simulink model "modelR2016bMAC"  (R2016b)
settings: Solver=VariableStepAuto  StartTime=0.0  StopTime=time  FixedStep=0.02  RelTol=1e-3  EnableMultiTasking=on
InitFcn:
  | m
StopFcn:
  | plotting
undefined symbols (not defined in the file): Aw, Awi, B, CurrentEnabled, D, E, e0, Eta0, g, Gi, Gpd, H, HiPAPpeaksEnabled, Is, Lambda, M, N, Omega, P0, path, Q, R, SensNoiseEnabled, T, tau_max, tau_min, Tb, WavesEnabled, x0
settings Model: Creator=Gaspar  LastModifiedBy=sbuadu
settings DataIOCC: LimitDataPoints=on  SaveFormat=Structure  SaveOutput=off  SaveTime=off
settings OptimizationCC: DefaultParameterBehavior=Inlined  LifeSpan=inf
settings DebuggingCC: UnderspecifiedInitializationDetection=Classic  MergeDetectMultiDrivingBlocksExec=none  SFUnexpectedBacktrackingDiag=warning  SFNoUnconditionalDefaultTransitionDiag=warning  SFExecutionAtInitializationDiag=none
settings GRTTargetCC: TargetLangStandard=C89/C90 (ANSI)
settings ConfigComp: CovMetricSettings=dw  CovHtmlReporting=on  CovSaveCumulativeToWorkspaceVar=on  CovSaveSingleToWorkspaceVar=on  CovExternalEMLEnable=off

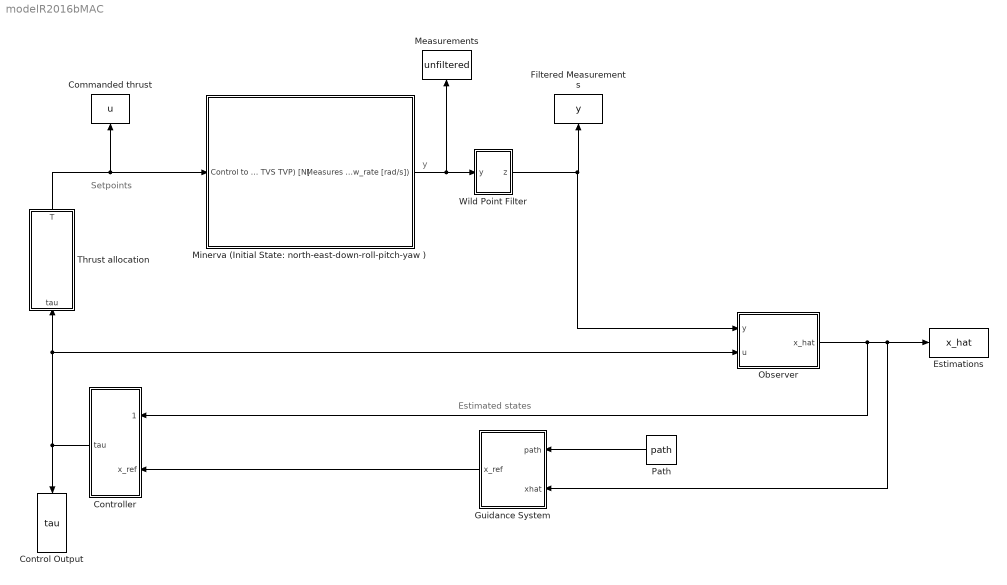
== system modelR2016bMAC ==
  note: Estimated states
  note: y
  note: Setpoints
  Commanded thrust : ToWorkspace  VariableName=u  SaveFormat=Timeseries  SampleTime=T
  Control Output : ToWorkspace  VariableName=tau  SaveFormat=Timeseries  SampleTime=-1
  Controller : Subsystem
  Estimations : ToWorkspace  VariableName=x_hat  SaveFormat=Timeseries  SampleTime=T
  Filtered Measurements : ToWorkspace  VariableName=y  SaveFormat=Timeseries  SampleTime=T
  Guidance System : Subsystem
  Measurements : ToWorkspace  VariableName=unfiltered  SaveFormat=Timeseries  SampleTime=T
  Minerva (Initial State: north-east-down-roll-pitch-yaw ) : Subsystem  mask{sfcnParam1=CurrentEnabled, sfcnParam2=Eta0, sfcnParam3=HiPAPpeaksEnabled, sfcnParam4=SensNoiseEnabled, sfcnParam5=WavesEnabled}
      mask prompts: sfcnParam1 "CurrentEnabled:"; sfcnParam2 "Eta0:"; sfcnParam3 "HiPAPpeaksEnabled:"; sfcnParam4 "SensNoiseEnabled:"; sfcnParam5 "WavesEnabled:"
      mask help: Simulink:masks:GenSFuncDesc_MD
      mask Help: eval('feval(''rtwprivate'',''rtwhelpview'',''rtw_sfcn_block'')');
      mask Display: image(imread(strcat(cd,'/ROVMinerva.jpg'),'jpg'),'center')
  Observer : Subsystem
  "Path " : Constant  Value=path  SampleTime=T
  "Thrust allocation " : Subsystem
  Wild Point Filter : Subsystem
  wires:
  Wild Point Filter/1(z) -> Observer/1(y), Filtered Measurements/1
  Minerva (Initial State: north-east-down-roll-pitch-yaw )/1(Measures (n[m] e[m] d[m] heading [rad] yaw_rate [rad/s])) -> Measurements/1, Wild Point Filter/1(y)
  "Thrust allocation "/1(T) -> Minerva (Initial State: north-east-down-roll-pitch-yaw )/1(Control to Thrusters (THS THP THL TVS TVP) [N]), Commanded thrust/1
  Controller/1(tau) -> Observer/2(u), "Thrust allocation "/1(tau), Control Output/1
  Observer/1(x_hat) -> Controller/1(x_hat), Guidance System/2("xhat "), Estimations/1
  "Path "/1 -> Guidance System/1(path)
  Guidance System/1(x_ref) -> Controller/2(x_ref)

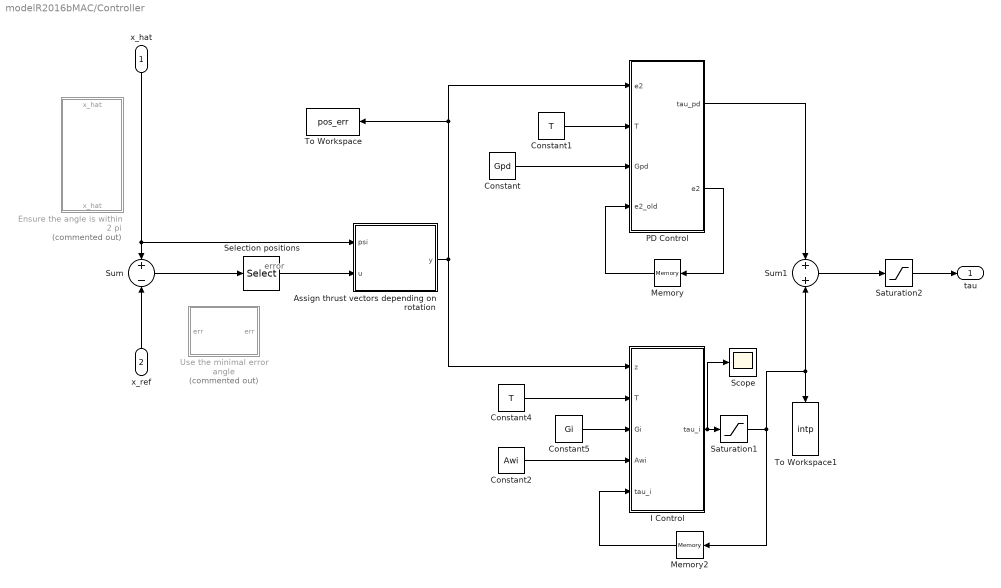
== system modelR2016bMAC/Controller ==
  note: error
  x_hat : Inport  PortDimensions=[20,1]  SampleTime=T
  x_ref : Inport  Port=2  PortDimensions=[20,1]  SampleTime=T
  Assign thrust vectors depending on rotation : MATLAB Function  TreatAsAtomicUnit=on
  Constant : Constant  Value=Gpd  SampleTime=T
  Constant1 : Constant  Value=T  SampleTime=T
  Constant2 : Constant  Value=Awi  SampleTime=T
  Constant4 : Constant  Value=T  SampleTime=T
  Constant5 : Constant  Value=Gi  SampleTime=T
  Ensure the angle is within 2 pi : MATLAB Function  Commented=on  TreatAsAtomicUnit=on
  I Control : MATLAB Function  TreatAsAtomicUnit=on
  Memory : Memory  X0=e0  InheritSampleTime=on
  Memory2 : Memory  X0=e0  InheritSampleTime=on
  PD Control : MATLAB Function  TreatAsAtomicUnit=on
  Saturation1 : Saturate  UpperLimit=Is*tau_max  LowerLimit=Is*tau_min
  Saturation2 : Saturate  UpperLimit=tau_max  LowerLimit=tau_min
  Scope : Scope
  Selection positions : Selector  InputPortWidth=20  IndexOptions=Index vector (dialog)  Indices=[9:12]  OutputSizes=1
  Sum : Sum  Inputs=+-
  Sum1 : Sum
  To Workspace : ToWorkspace  VariableName=pos_err  SaveFormat=Timeseries  SampleTime=T
  To Workspace1 : ToWorkspace  VariableName=intp  SaveFormat=Timeseries  SampleTime=T
  Use the minimal error angle : MATLAB Function  Commented=on  TreatAsAtomicUnit=on
  tau : Outport  PortDimensions=[4,1]  SampleTime=T
  wires:
  x_ref/1 -> Sum/2
  Constant/1 -> PD Control/3(Gpd)
  PD Control/2(e2) -> Memory/1
  Memory/1 -> PD Control/4(e2_old)
  Constant1/1 -> PD Control/2(T)
  Sum/1 -> Selection positions/1
  Constant4/1 -> I Control/2(T)
  Constant5/1 -> I Control/3(Gi)
  I Control/1(tau_i) -> Scope/1, Saturation1/1
  Memory2/1 -> I Control/5("tau_i ")
  Constant2/1 -> I Control/4(Awi)
  Saturation1/1 -> Memory2/1, Sum1/2, To Workspace1/1
  PD Control/1(tau_pd) -> Sum1/1
  Sum1/1 -> Saturation2/1
  Selection positions/1 -> Assign thrust vectors depending on rotation/2(u)
  x_hat/1 -> Assign thrust vectors depending on rotation/1(psi), Sum/1
  Assign thrust vectors depending on rotation/1(y) -> I Control/1(z), To Workspace/1, PD Control/1("e2 ")
  Saturation2/1 -> tau/1

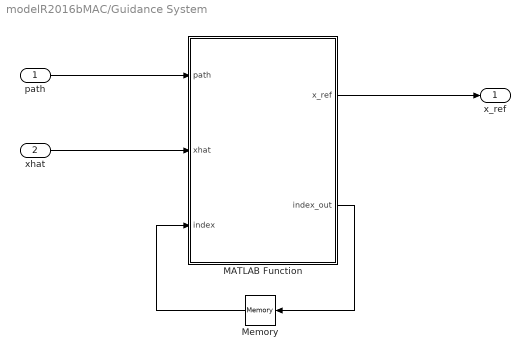
== system modelR2016bMAC/Guidance System ==
  path : Inport  SampleTime=T
  "xhat " : Inport  Port=2  SampleTime=T
  MATLAB Function : MATLAB Function  TreatAsAtomicUnit=on
  Memory : Memory  X0=1  InheritSampleTime=on
  x_ref : Outport  PortDimensions=[20,1]  SampleTime=T
  wires:
  path/1 -> MATLAB Function/1(path)
  MATLAB Function/1(x_ref) -> x_ref/1
  MATLAB Function/2(index_out) -> Memory/1
  Memory/1 -> MATLAB Function/3(index)
  "xhat "/1 -> MATLAB Function/2(xhat)

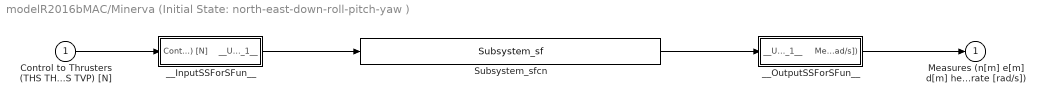
== system modelR2016bMAC/Minerva (Initial State: north-east-down-roll-pitch-yaw ) ==
  Control to Thrusters (THS THP THL TVS TVP) [N] : Inport  OutDataTypeStr=double  PortDimensions=5  SampleTime=0.2
  Subsystem_sfcn : S-Function  FunctionName=Subsystem_sf  Parameters=sfcnParam1, sfcnParam2, sfcnParam3, sfcnParam4, sfcnParam5  SFunctionModules=""  SFunctionDeploymentMode=off  EnableBusSupport=off  SFcnStateName=DWORK0  mask{rtw_sf_name=Subsystem_sf, showVar=off, sfcnParam1=sfcnParam1, sfcnParam2=sfcnParam2, sfcnParam3=sfcnParam3, sfcnParam4=sfcnParam4, sfcnParam5=sfcnParam5}
      mask prompts: rtw_sf_name "Simulink:masks:GenSFuncName_MP"; showVar "Simulink:masks:GenSFuncShowModuleList_MP"; sfcnParam1 "CurrentEnabled:"; sfcnParam2 "Eta0:"; sfcnParam3 "HiPAPpeaksEnabled:"; sfcnParam4 "SensNoiseEnabled:"; sfcnParam5 "WavesEnabled:"
      mask help: Simulink:masks:GenSFuncDesc_MD
      mask init:
      | displist = '';
      | if ~strcmp(get_param(gcb, 'FunctionName'), rtw_sf_name);
      |   set_param(gcb, 'FunctionName', rtw_sf_name);
      | end
      | % Check if we are generating code
      | rtw_mode = false;
      | if strcmpi(get_param(bdroot(gcb),'SimulationStatus'),'Initializing')
      | 	rtw_mode = strcmpi(get_param(bdroot(gcb),'BuildingRTWCode'),'on') && ...
      | 		~strcmpi(get_param(bdroot(gcb),'TargetStyle'),'SimulationTarget');
      | end
      | if showVar || rtw_mode
      | 	if exist('rtwsfunc') == 2 | exist('rtwsfunc') == 6
      | 		tmplist = rtwsfunc(rtw_sf_name,gcb);
      | 		tmplist = DAStudio.message('Simulink:masks:GenSFuncListOfModules_IC', tmplist);
      | 	elseif showVar
      | 		tmplist1 = DAStudio.message('Simulink:masks:GenSFuncListOfModules_IC', '');
      |         tmplist2 = DAStudio.message('Simulink:masks:GenSFuncNotLicensed_IC');
      |         tmplist = [tmplist1 tmplist2];
      |  	end
      | end
      | if showVar
      |   displist = tmplist;
      | end
      settings: SFcnIsStateOwnerBlock=on
      settings: CopyFcn=|
      | if ~strcmp(get_param(gcb,'Linkstatus'),'none') && ...
      | ~strcmp(get_param(gcb,'Linkstatus'),'implicit')
      |   set_param(gcb,'LinkStatus','none');
      | end
      mask Help: eval('feval(''rtwprivate'',''rtwhelpview'',''rtw_sfcn_block'')');
      mask Display:
      | port_label('input',1,'Control to Thrusters (THS THP THL TVS TVP) [N]');
      | port_label('output',1,'Measures (n[m] e[m] d[m] heading [rad] yaw_rate [rad/s])');
  __InputSSForSFun__ : Subsystem
  __OutputSSForSFun__ : Subsystem
  Measures (n[m] e[m] d[m] heading [rad] yaw_rate [rad/s]) : Outport  OutDataTypeStr=double  PortDimensions=5  SampleTime=[0.20000000000000001,0]
  wires:
  Control to Thrusters (THS THP THL TVS TVP) [N]/1 -> __InputSSForSFun__/1(Control to Thrusters (THS THP THL TVS TVP) [N])
  __InputSSForSFun__/1(__UniqueOutportName__1__) -> Subsystem_sfcn/1
  Subsystem_sfcn/1 -> __OutputSSForSFun__/1(__UniqueInportName__1__)
  __OutputSSForSFun__/1(Measures (n[m] e[m] d[m] heading [rad] yaw_rate [rad/s])) -> Measures (n[m] e[m] d[m] heading [rad] yaw_rate [rad/s])/1

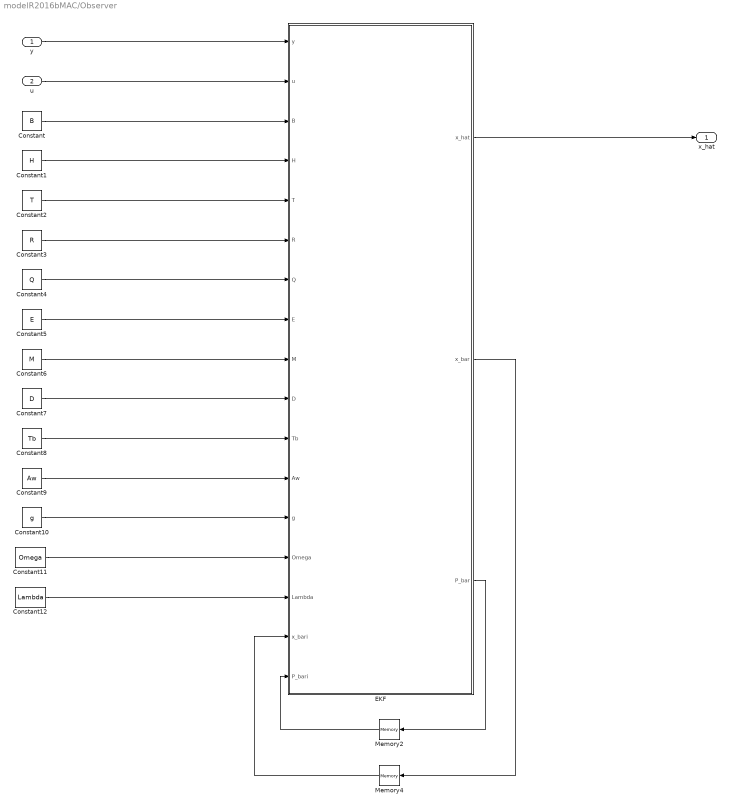
== system modelR2016bMAC/Observer ==
  y : Inport  PortDimensions=[5,1]
  u : Inport  Port=2  PortDimensions=[4,1]
  Constant : Constant  Value=B  SampleTime=T
  Constant1 : Constant  Value=H  SampleTime=T
  Constant10 : Constant  Value=g  SampleTime=T
  Constant11 : Constant  Value=Omega  SampleTime=T
  Constant12 : Constant  Value=Lambda  SampleTime=T
  Constant2 : Constant  Value=T  SampleTime=T
  Constant3 : Constant  Value=R  SampleTime=T
  Constant4 : Constant  Value=Q  SampleTime=T
  Constant5 : Constant  Value=E  SampleTime=T
  Constant6 : Constant  Value=M  SampleTime=T
  Constant7 : Constant  Value=D  SampleTime=T
  Constant8 : Constant  Value=Tb  SampleTime=T
  Constant9 : Constant  Value=Aw  SampleTime=T
  EKF : MATLAB Function  TreatAsAtomicUnit=on
  Memory2 : Memory  X0=P0  InheritSampleTime=on
  Memory4 : Memory  X0=x0  InheritSampleTime=on
  x_hat : Outport  PortDimensions=[20,1]
  wires:
  y/1 -> EKF/1(y)
  u/1 -> EKF/2(u)
  Constant/1 -> EKF/3(B)
  Constant1/1 -> EKF/4(H)
  Constant2/1 -> EKF/5(T)
  EKF/3(P_bar) -> Memory2/1
  Memory2/1 -> EKF/17(P_bari)
  EKF/1(x_hat) -> x_hat/1
  EKF/2(x_bar) -> Memory4/1
  Memory4/1 -> EKF/16(x_bari)
  Constant3/1 -> EKF/6(R)
  Constant4/1 -> EKF/7(Q)
  Constant5/1 -> EKF/8(E)
  Constant9/1 -> EKF/12(Aw)
  Constant6/1 -> EKF/9(M)
  Constant7/1 -> EKF/10(D)
  Constant8/1 -> EKF/11(Tb)
  Constant10/1 -> EKF/13(g)
  Constant12/1 -> EKF/15(Lambda)
  Constant11/1 -> EKF/14(Omega)

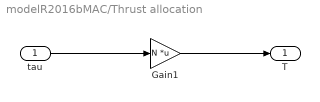
== system modelR2016bMAC/Thrust allocation  ==
  tau : Inport  SampleTime=T
  Gain1 : Gain  Gain=N  Multiplication=Matrix(K*u)
  T : Outport  SampleTime=T
  wires:
  tau/1 -> Gain1/1
  Gain1/1 -> T/1

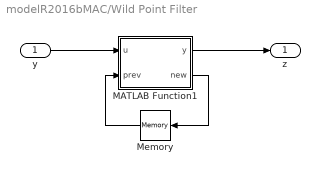
== system modelR2016bMAC/Wild Point Filter ==
  y : Inport
  MATLAB Function1 : MATLAB Function  TreatAsAtomicUnit=on
  Memory : Memory  InheritSampleTime=on
  z : Outport
  wires:
  y/1 -> MATLAB Function1/1(u)
  Memory/1 -> MATLAB Function1/2(prev)
  MATLAB Function1/2(new) -> Memory/1
  MATLAB Function1/1(y) -> z/1

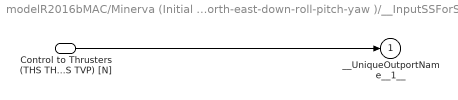
== system modelR2016bMAC/Minerva (Initial State: north-east-down-roll-pitch-yaw )/__InputSSForSFun__ ==
  Control to Thrusters (THS THP THL TVS TVP) [N] : Inport  OutDataTypeStr=double  PortDimensions=5  SampleTime=0.2
  __UniqueOutportName__1__ : Outport
  wires:
  Control to Thrusters (THS THP THL TVS TVP) [N]/1 -> __UniqueOutportName__1__/1

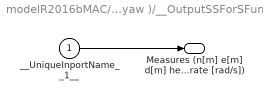
== system modelR2016bMAC/Minerva (Initial State: north-east-down-roll-pitch-yaw )/__OutputSSForSFun__ ==
  __UniqueInportName__1__ : Inport
  Measures (n[m] e[m] d[m] heading [rad] yaw_rate [rad/s]) : Outport  OutDataTypeStr=double  PortDimensions=5  SampleTime=[0.20000000000000001,0]
  wires:
  __UniqueInportName__1__/1 -> Measures (n[m] e[m] d[m] heading [rad] yaw_rate [rad/s])/1

== matlab function modelR2016bMAC/Wild Point Filter/MATLAB Function1 ==
  data: u input; y output; prev input; new output
function [y, new] = fcn(u, prev)
y = u;
elems = 11;
new = zeros(5,elems);
if numel(prev) == 1
    new = [repmat(zeros(5,1), 1, elems-1), u];
else
    new = prev;
end
avg = mean(diff(new'))'+new(:,end);

power = 4;
for i = 1:2
    if u(i) < avg(i) - power || u(i) > avg(i) + power
        y(i) = avg(i);
        u(i) = y(i);
    end
end
%{
last = interp1(new(2,:),1:elems+1);
for i = 2:2
if u(i) < last(end) - 4 || u(i) > last(end) + 4
    y(i) = last(end);
    u(i) = y(i);
end
end
%}

new = [prev(:,2:elems), u];

== matlab function modelR2016bMAC/Controller/Assign thrust vectors depending on rotation ==
  data: psi input; u input; y output
function y = thrustlocal(psi, u)
psi = psi(12);
J = @(psi) [cos(psi) -sin(psi) 0 0;
            sin(psi) cos(psi)  0 0;
            0        0         1 0;
            0        0         0 1];
y = transpose(J(psi))*u;

== matlab function modelR2016bMAC/Controller/PD Control ==
  data: e2 input; T input; tau_pd output; Gpd input; e2 output; e2_old input
function [tau_pd, e2] = pd(e2, T, Gpd, e2_old)
% The change in position error
e1 = (e2 - e2_old)/T;

% Calculating control action using gain matrix
e_tot = [e2' e1']';
tau_pd = -Gpd*e_tot;

== matlab function modelR2016bMAC/Observer/EKF ==
  data: y input; u input; x_hat output; x_bar output; B input; H input; T input; R input; Q input; E input; M input; D input; Tb input; Aw input; g input; Omega input; Lambda input; x_bari input; P_bari input; P_bar output
function [x_hat, x_bar, P_bar] = ekf(y, u, B, H, T, R, Q, E, M, D, Tb, Aw, g, Omega, Lambda, x_bari, P_bari)
    % Corrector
    y = y(1:4);
    K = P_bari*H'*inv(H*P_bari*H'+R);
    P_hat = (eye(20)-K*H)*P_bari*(eye(20)-K*H)'+K*R*K';
    x_hat = x_bari + K*(y-H*x_bari);
    
    J = @(psi) [cos(psi) -sin(psi) 0 0;
                sin(psi) cos(psi) 0 0;
                0 0 1 0;
                0 0 0 1];
    
    xi = x_hat(1:8);
    eta = x_hat(9:12);
    b = x_hat(13:16);
    nu = x_hat(17:20);
    psi = eta(4);
    f = [Aw*xi;
         J(psi)*nu;
         -inv(Tb)*b;
         -inv(M)*D*nu - inv(M)*g + inv(M)*J(psi)'*b];     
    
    Phi = [1, 0, 0, 0, T, 0, 0, 0, 0, 0, 0, 0, 0, 0, 0, 0, 0, 0, 0, 0;
           0, 1, 0, 0, 0, T, 0, 0, 0, 0, 0, 0, 0, 0, 0, 0, 0, 0, 0, 0;
           0, 0, 1, 0, 0, 0, T, 0, 0, 0, 0, 0, 0, 0, 0, 0, 0, 0, 0, 0;
           0, 0, 0, 1, 0, 0, 0, T, 0, 0, 0, 0, 0, 0, 0, 0, 0, 0, 0, 0;
           -Omega(1,1)^2*T, 0, 0, 0, -2*Lambda(1,1)*Omega(1,1)*T + 1, 0, 0, 0, 0, 0, 0, 0, 0, 0, 0, 0, 0, 0, 0, 0;
           0, -Omega(2,2)^2*T, 0, 0, 0, -2*Lambda(2,2)*Omega(2,2)*T + 1, 0, 0, 0, 0, 0, 0, 0, 0, 0, 0, 0, 0, 0, 0;
           0, 0, -Omega(3,3)^2*T, 0, 0, 0, -2*Lambda(3,3)*Omega(3,3)*T + 1, 0, 0, 0, 0, 0, 0, 0, 0, 0, 0, 0, 0, 0;
           0, 0, 0, -Omega(4,4)^2*T, 0, 0, 0, -2*Lambda(4,4)*Omega(4,4)*T + 1, 0, 0, 0, 0, 0, 0, 0, 0, 0, 0, 0, 0;
           0, 0, 0, 0, 0, 0, 0, 0, 1, 0, 0, 0, 0, 0, 0, 0, T*cos(psi), -T*sin(psi), 0, 0;
           0, 0, 0, 0, 0, 0, 0, 0, 0, 1, 0, 0, 0, 0, 0, 0, T*sin(psi), T*cos(psi), 0, 0;
           0, 0, 0, 0, 0, 0, 0, 0, 0, 0, 1, 0, 0, 0, 0, 0, 0, 0, T, 0;
           0, 0, 0, 0, 0, 0, 0, 0, 0, 0, 0, 1, 0, 0, 0, 0, 0, 0, 0, T;
           0, 0, 0, 0, 0, 0, 0, 0, 0, 0, 0, 0, -T/Tb(1,1) + 1, 0, 0, 0, 0, 0, 0, 0;
           0, 0, 0, 0, 0, 0, 0, 0, 0, 0, 0, 0, 0, -T/Tb(2,2) + 1, 0, 0, 0, 0, 0, 0;
           0, 0, 0, 0, 0, 0, 0, 0, 0, 0, 0, 0, 0, 0, -T/Tb(3,3) + 1, 0, 0, 0, 0, 0;
           0, 0, 0, 0, 0, 0, 0, 0, 0, 0, 0, 0, 0, 0, 0, -T/Tb(4,4) + 1, 0, 0, 0, 0;
           0, 0, 0, 0, 0, 0, 0, 0, 0, 0, 0, 0, T*cos(psi)/M(1,1),-T*sin(psi)/M(1,1), 0, 0, -D(1,1)*T/M(1,1) + 1, 0, 0, 0;
           0, 0, 0, 0, 0, 0, 0, 0, 0, 0, 0, 0, T*sin(psi)/M(2,2),T*cos(psi)/M(2,2), 0, 0, 0, -D(2,2)*T/M(2,2) + 1, 0, 0;
           0, 0, 0, 0, 0, 0, 0, 0, 0, 0, 0, 0, 0, 0, T/M(3,3), 0, 0, 0,-D(3,3)*T/M(3,3) + 1, 0;
           0, 0, 0, 0, 0, 0, 0, 0, 0, 0, 0, 0, 0, 0, 0, T/M(4,4), 0, 0, 0,-D(4,4)*T/M(4,4) + 1];
    
    
    % Predictor
    P_bar = Phi*P_hat*Phi' + T^2*E*Q*E';
    x_bar = x_hat + T*(f + B*u);
end

== matlab function modelR2016bMAC/Controller/I Control ==
  data: z input; tau_i output; T input; Gi input; Awi input; tau_i input
function tau_i = integral(z, T, Gi, Awi, tau_i)
%{
    % Calculating area using trapezoid rule
    area = T*(pos_err-pos_err_in)/2;

    % Adding the area to the integral sum
    integrals_out = integrals + area;

    % Calculation integral control
    tau_i = -Gi*integrals_out;

    pos_err_out = pos_err_in;
%}
% Euler method in time
tau_i = T*(Awi*tau_i + Gi*z) + tau_i;

== matlab function modelR2016bMAC/Controller/Ensure the angle is within 2 pi ==
  data: x_hat input; x_hat output
function x_hat = anglelimit(x_hat)
% x_hat(12) = wrapTo2Pi(x_hat(12));
x_hat(12) = mod(x_hat(12), 2*pi);

== matlab function modelR2016bMAC/Controller/Use the minimal error angle ==
  data: err input; err output
function err = errorangle(err)
if 2*pi - err(12) < err(12)
    err(12) = 2*pi - err(12);
end

== matlab function modelR2016bMAC/Guidance System/MATLAB Function ==
  data: path input; x_ref output; xhat input; index input; index_out output
function [x_ref, index_out]= fcn(path, xhat, index)

setpoint = path(:,index);   %defining the current setpoint
diffs = abs(path(1:3,index) - xhat(9:11));  %finding the distance from Minerva to current setpoint
diff_psi = abs(path(4,index) - xhat(12));   %finding the deviation between desired heading and actuall heading

if index+1 <= size(path, 2)     % checking that the are more way points 
    if norm(diffs) < 5 && diff_psi < 10*pi/180 %acceptance critearia 
        index_out = index + 1;
        setpoint = path(:, index_out);
    end
end

x_ref = zeros(20,1);
x_ref(9:12) = setpoint;     %setting a setpoint for the controller 

end
